simulink model "sFunctionLibrary_create_desRN_Harness"  (R2025b)
settings: Solver=FixedStepAuto  StartTime=1  StopTime=101  FixedStep=1  RelTol=1e-3
settings Model: Creator=AdamY  LastModifiedBy=AdamY

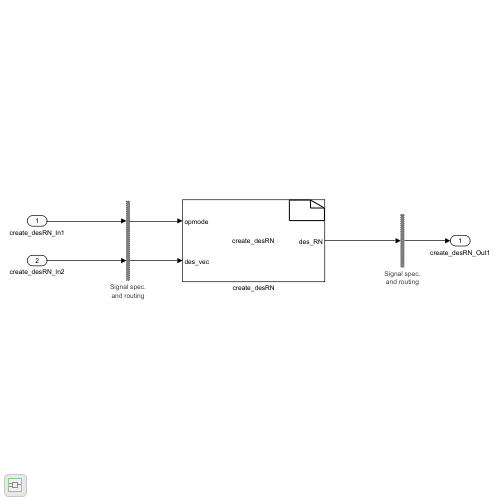
[thumbnail: Simulink's stored preview of the top-level diagram]
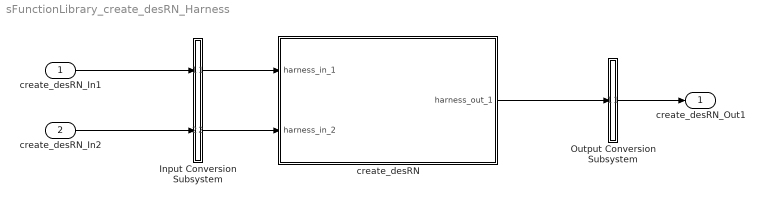
== system sFunctionLibrary_create_desRN_Harness ==
  create_desRN_In1 : Inport
  create_desRN_In2 : Inport  Port=2
  Input Conversion Subsystem : Subsystem  Tag=__SLT_ICS__  Description=|
      | Signal spec.
      | and routing
      settings: AttributesFormatString=%<Description>
  Output Conversion Subsystem : Subsystem  Tag=__SLT_OCS__  Description=|
      | Signal spec.
      | and routing
      settings: AttributesFormatString=%<Description>
  create_desRN : Subsystem  Tag=__SL_testing_harness_stub_
  create_desRN_Out1 : Outport
  wires:
  create_desRN_In1/1 -> Input Conversion Subsystem/1(Inport_1)
  create_desRN_In2/1 -> Input Conversion Subsystem/2(Inport_2)
  Output Conversion Subsystem/1(Outport_1) -> create_desRN_Out1/1
  Input Conversion Subsystem/1(Outport_1) -> create_desRN/1(harness_in_1)
  Input Conversion Subsystem/2(Outport_2) -> create_desRN/2(harness_in_2)
  create_desRN/1(harness_out_1) -> Output Conversion Subsystem/1(Inport_1)

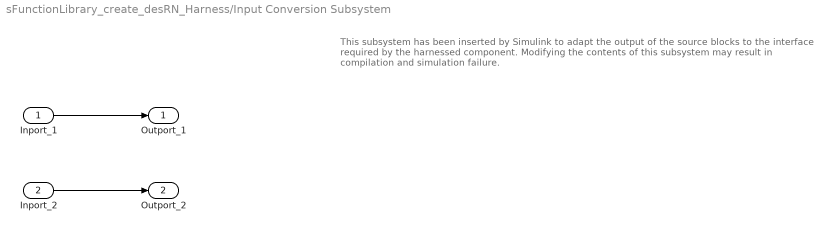
== system sFunctionLibrary_create_desRN_Harness/Input Conversion Subsystem ==
  note: This subsystem has been inserted by Simulink to adapt the output of the source blocks to the interface required by the harnessed component.
      |  Modifying the contents of this subsystem may result in compilation and simulation failure.
  Inport_1 : Inport
  Inport_2 : Inport  Port=2
  Outport_1 : Outport
  Outport_2 : Outport  Port=2
  wires:
  Inport_1/1 -> Outport_1/1
  Inport_2/1 -> Outport_2/1

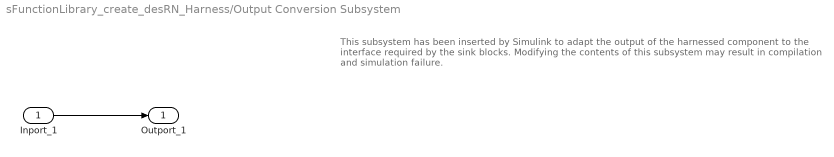
== system sFunctionLibrary_create_desRN_Harness/Output Conversion Subsystem ==
  note: This subsystem has been inserted by Simulink to adapt the output of the harnessed component to the interface required by the sink blocks.
      |  Modifying the contents of this subsystem may result in compilation and simulation failure.
  Inport_1 : Inport
  Outport_1 : Outport
  wires:
  Inport_1/1 -> Outport_1/1

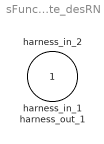
== system sFunctionLibrary_create_desRN_Harness/create_desRN ==
  harness_in_1 : Inport
  harness_in_2 : Inport  Port=2
  harness_out_1 : Outport
